simulink model "ScriptDemo"  (R2022b)
settings: configuration reference "TmVcThermal_Configuration_sub" (kept outside this file)
undefined symbols (not defined in the file): aaaa, bbbb, cTmComprCtrl_D_u8HvacFlowTable_db, cTmComprCtrl_D_u8HvacFlowTable_sw, cTmComprCtrl_n_i16ChillCmpIMax, cTmComprCtrl_n_i16ChillCmpIMin, cTmComprCtrl_n_i16ChillCmpIMin666, cTmComprCtrl_n_i16ChillCmpPMax, cTmComprCtrl_n_i16ChillCmpPMin, cTmComprCtrl_n_i16CmpChillCoolRpmKiMax, cTmComprCtrl_n_i16CmpChillCoolRpmKiMin, cTmComprCtrl_n_i16CmpChillCoolRpmKpMax, cTmComprCtrl_n_i16CmpChillCoolRpmKpMin, cTmComprCtrl_n_i16CmpCoolRpmKiMax, cTmComprCtrl_n_i16CmpCoolRpmKiMin, cTmComprCtrl_n_i16CmpCoolRpmKpMax, cTmComprCtrl_n_i16CmpCoolRpmKpMin, cTmComprCtrl_n_i16SM4CmpHeatKiMax, cTmComprCtrl_n_i16SM4CmpHeatKiMin, cTmComprCtrl_n_i16SM4CmpHeatKpMax, cTmComprCtrl_n_i16SM4CmpHeatKpMin, cTmComprCtrl_n_i16SM5CmpHeatKiMax, cTmComprCtrl_n_i16SM5CmpHeatKiMin, cTmComprCtrl_n_i16SM5CmpHeatKpMax, cTmComprCtrl_n_i16SM5CmpHeatKpMin, cTmComprCtrl_n_i16SM6CmpHeatKiMax, cTmComprCtrl_n_i16SM6CmpHeatKiMin, cTmComprCtrl_n_i16SM6CmpHeatKpMax, cTmComprCtrl_n_i16SM6CmpHeatKpMin, cTmComprCtrl_n_u16CmpMaxSpdFanFltLimt, cTmComprCtrl_n_u16CmpMaxSpdLoSidePFltLimt, cTmComprCtrl_n_u16CmpMaxSpdSensorFltLimt, cTmComprCtrl_n_u16CompMinRpm, cTmComprCtrl_n_u16CompRpmIncThres, cTmComprCtrl_t_u16BattCooltFFPeriod, cTmComprCtrl_t_u16BattCooltPIPeriod, cTmComprCtrl_t_u16CmpCoolFFPeriod, cTmComprCtrl_t_u16CmpCoolPIPeriod, cTmComprCtrl_t_u16CoolCmpChillFFPeriod, cTmComprCtrl_t_u16CoolCmpChillPIPeriod, cTmComprCtrl_t_u16SM4CmpHeatFFPeriod, cTmComprCtrl_t_u16SM4CmpHeatPIPeriod, cTmComprCtrl_t_u16SM5CmpHeatFFPeriod, cTmComprCtrl_t_u16SM5CmpHeatPIPeriod, cTmComprCtrl_t_u16SM6CmpHeatFFPeriod, cTmComprCtrl_t_u16SM6CmpHeatPIPeriod, cTmComprCtrl_Te_EvapClearInteg, cTmComprCtrl_Te_i16HpReqTempSaturoffset, cTmComprCtrl_Te_i16SatLpReplaceDiff, cTmComprCtrl_Te_i16SM3BatDiffStartEvapDecOffset, cTmComprCtrl_Te_i16SM3EvapLo, cTmComprCtrl_Te_i16SM3TBatDiffEntEvapDecOffset, cTmComprCtrl_Te_i16SM3TBatDiffEntEvapDecOffsetQuit, cTmComprCtrl_Te_s32ErrCmpChillPIContinueCoolH, cTmComprCtrl_Te_s32ErrCmpChillPIContinueCoolL, cTmComprCtrl_Te_s32ErrCmpPIContinueChillH, cTmComprCtrl_Te_s32ErrCmpPIContinueChillL, cTmComprCtrl_Te_s32ErrCmpPIContinueCoolH, cTmComprCtrl_Te_s32ErrCmpPIContinueCoolL, cTmComprCtrl_Te_s32ErrCmpPIContinueHeatH ... (+398)
libraries: simulink x782, PCMULib x640, simulink_need_slupdate x4
(part 13 of 41)

== system ScriptDemo/Create/createMerge/After/SM2SM22 ==
  note: 1: 非热泵
      | 2：热泵
  sTmSigProces_Te_s32EvapFanReqRamp : Inport  OutDataTypeStr=single
  sTmDiag_D_u8TeEvapFltSt : Inport  Port=2  OutDataTypeStr=uint8
  sTmIn_D_u8HeatPump : Inport  Port=3  OutDataTypeStr=uint8
  sTmSigProces_Te_s32TAmb : Inport  Port=4  OutDataTypeStr=single
  sTmIn_X_s32ClimtRcirc : Inport  Port=5  OutDataTypeStr=single
  sTmComprCtrl_D_u8HvacFlowLevel : Inport  Port=6  OutDataTypeStr=uint8
  sTmSigProces_Te_s32EvapFanFilter : Inport  Port=7  OutDataTypeStr=single
  sTmSigProces_Te_s32SatLp : Inport  Port=8  OutDataTypeStr=single
  xTmComprCtrl_B_CompOnReqCompOn : Inport  Port=9  OutDataTypeStr=boolean
  yTmRefriModeMgr_B_CoolModeInCycle : Inport  Port=10  OutDataTypeStr=boolean
  yTmRefriModeMgr_B_CoolOCRMode : Inport  Port=11  OutDataTypeStr=boolean
  sTmSigProces_Pw_i16ReqPwrForCool : Inport  Port=12  OutDataTypeStr=int16
  Action Port : ActionPort
  1-D Lookup Table : Lookup_n-D  NumberOfTableDimensions=1  BreakpointsForDimension1=tTmComprCtrl_n_i16CmpCoolRpmKiMin_X  BreakpointsForDimension1DataTypeStr=Inherit: Inherit from 'Breakpoint data'  Table=tTmComprCtrl_n_i16CmpCoolRpmKiMin  TableDataTypeStr=Inherit: Inherit from 'Table data'  ExtrapMethod=Clip  InternalRulePriority=Speed  OutDataTypeStr=Inherit: Inherit via back propagation  RndMeth=Simplest  InputSameDT=off
  1-D Lookup Table1 : Lookup_n-D  NumberOfTableDimensions=1  BreakpointsForDimension1=tTmComprCtrl_n_i16CmpCoolRpmKiMax_X  BreakpointsForDimension1DataTypeStr=Inherit: Inherit from 'Breakpoint data'  Table=tTmComprCtrl_n_i16CmpCoolRpmKiMax  TableDataTypeStr=Inherit: Inherit from 'Table data'  ExtrapMethod=Clip  InternalRulePriority=Speed  OutDataTypeStr=Inherit: Inherit via back propagation  RndMeth=Simplest  InputSameDT=off
  Compare To Constant1 : simulink/Logic and Bit Operations/Compare To Constant  relop===  const=2  OutDataTypeStr=boolean
  Constant : Constant  Value=cTmComprCtrl_n_i16CmpCoolRpmKpMax  OutDataTypeStr=int16
  Constant3 : Constant  Value=cTmComprCtrl_t_u16CmpCoolPIPeriod  OutDataTypeStr=uint16
  Constant4 : Constant  Value=cTmComprCtrl_n_i16CmpCoolRpmKpMin  OutDataTypeStr=int16
  Constant5 : Constant  Value=cTmComprCtrl_Te_s32ErrCmpPIContinueCoolH  OutDataTypeStr=single
  Constant6 : Constant  Commented=on  Value=cTmComprCtrl_n_i16CmpCoolRpmKiMax  OutDataTypeStr=int16
  Constant7 : Constant  Value=cTmComprCtrl_Te_s32ErrCmpPIContinueCoolL  OutDataTypeStr=single
  Constant8 : Constant  Commented=on  Value=cTmComprCtrl_n_i16CmpCoolRpmKiMin  OutDataTypeStr=int16
  Constant9 : Constant  Value=cTmComprCtrl_n_u16CompMinRpm
  ID26239_SM2Error : Subsystem
  ID26267_SM2FF : Subsystem
  Logical Operator : Logic  AllPortsSameDT=off  OutDataTypeStr=boolean
  Logical Operator2 : Logic  Operator=NOT  AllPortsSameDT=off  OutDataTypeStr=boolean
  SM2FFEnable : Subsystem
  SM2_Ki : Subsystem
  SM2_Kp : Subsystem
  rSM2SM22_n_u16DisOverrideValue : Outport  OutDataTypeStr=uint16
  rSM2SM22_t_u16PIPeriod : Outport  Port=2  OutDataTypeStr=uint16
  rSM2SM22_Te_s32UpErrStop : Outport  Port=3  OutDataTypeStr=single
  rSM2SM22_n_u16ComprRpmFF : Outport  Port=4  OutDataTypeStr=uint16
  rSM2SM22_n_u16ComprRpmKp : Outport  Port=5  OutDataTypeStr=uint16
  rSM2SM22_n_u16ComprRpmKi : Outport  Port=6  OutDataTypeStr=uint16
  rSM2SM22_Te_s32LowErrStop : Outport  Port=7  OutDataTypeStr=single
  rSM2SM22_n_i16KpUpLimit : Outport  Port=8  OutDataTypeStr=int16
  rSM2SM22_n_i16KpLowLimit : Outport  Port=9  OutDataTypeStr=int16
  rSM2SM22_n_i16KiUpLimit : Outport  Port=10  OutDataTypeStr=int16
  rSM2SM22_n_i16KiLowLimit : Outport  Port=11  OutDataTypeStr=int16
  xSM2SM22_B_Enable : Outport  Port=12  OutDataTypeStr=boolean
  rSM2SM22_Te_s32TempError : Outport  Port=13  OutDataTypeStr=single
  wires:
  sTmSigProces_Te_s32EvapFanReqRamp/1 -> [sTmSigProces_Te_s32EvapFanReqRamp]
  sTmDiag_D_u8TeEvapFltSt/1 -> [sTmDiag_D_u8TeEvapFltSt]
  sTmIn_D_u8HeatPump/1 -> [sTmIn_D_u8HeatPump]
  sTmSigProces_Te_s32TAmb/1 -> [sTmSigProces_Te_s32TAmb]
  sTmIn_X_s32ClimtRcirc/1 -> [sTmIn_X_s32ClimtRcirc]
  sTmComprCtrl_D_u8HvacFlowLevel/1 -> [sTmComprCtrl_D_u8HvacFlowLevel]
  sTmSigProces_Te_s32EvapFanFilter/1 -> [sTmSigProces_Te_s32EvapFanFilter]
  sTmSigProces_Te_s32SatLp/1 -> [sTmSigProces_Te_s32SatLp]
  xTmComprCtrl_B_CompOnReqCompOn/1 -> [xTmComprCtrl_B_CompOnReqCompOn]
  yTmRefriModeMgr_B_CoolModeInCycle/1 -> [yTmRefriModeMgr_B_CoolModeInCycle]
  [sTmSigProces_Te_s32EvapFanReqRamp] -> ID26267_SM2FF/1(sTmSigProces_Te_s32EvapFanReqRamp)
  [sTmSigProces_Te_s32TAmb] -> ID26267_SM2FF/2(sTmSigProces_Te_s32TAmb)
  [sTmIn_X_s32ClimtRcirc] -> ID26267_SM2FF/3(sTmIn_X_s32ClimtRcirc)
  [sTmComprCtrl_D_u8HvacFlowLevel] -> ID26267_SM2FF/4(sTmComprCtrl_D_u8HvacFlowLevel)
  [rTmComprCtrl_Te_s32TempError] -> SM2_Ki/1(rTmComprCtrl_Te_s32TempError)
  [sTmSigProces_Te_s32TAmb] -> SM2_Ki/2(sTmSigProces_Te_s32TAmb)
  [sTmIn_X_s32ClimtRcirc] -> SM2_Ki/3(sTmIn_X_s32ClimtRcirc)
  [sTmComprCtrl_D_u8HvacFlowLevel] -> SM2_Ki/4(sTmComprCtrl_D_u8HvacFlowLevel)
  [rTmComprCtrl_Te_s32TempError] -> SM2_Kp/1(rTmComprCtrl_Te_s32TempError)
  [sTmSigProces_Te_s32TAmb] -> SM2_Kp/2(sTmSigProces_Te_s32TAmb)
  [sTmIn_X_s32ClimtRcirc] -> SM2_Kp/3(sTmIn_X_s32ClimtRcirc)
  [sTmComprCtrl_D_u8HvacFlowLevel] -> SM2_Kp/4(sTmComprCtrl_D_u8HvacFlowLevel)
  [sTmSigProces_Te_s32EvapFanReqRamp] -> ID26239_SM2Error/1(sTmSigProces_Te_s32EvapFanReqRamp)
  [sTmDiag_D_u8TeEvapFltSt] -> ID26239_SM2Error/2(sTmDiag_D_u8TeEvapFltSt)
  [sTmSigProces_Te_s32EvapFanFilter] -> ID26239_SM2Error/3(sTmSigProces_Te_s32EvapFanFilter)
  [sTmSigProces_Te_s32SatLp] -> ID26239_SM2Error/4(sTmSigProces_Te_s32SatLp)
  SM2FFEnable/1(SM2FFEnable_B_SM2FFEnable) -> [SM2FFEnable_B_SM2FFEnable]
  [xTmComprCtrl_B_CompOnReqCompOn] -> SM2FFEnable/1(xTmComprCtrl_B_CompOnReqCompOn)
  [SM2FFEnable_B_SM2FFEnable] -> ID26267_SM2FF/Enable
  ID26239_SM2Error/1(rTmComprCtrl_Te_s32TempError) -> [rTmComprCtrl_Te_s32TempError]
  ID26267_SM2FF/1(SM2FF) -> [rTmComprCtrl_n_u16ComprRpmFF]
  SM2_Kp/1(SM2Kp) -> [rTmComprCtrl_n_u16ComprRpmKp]
  SM2_Ki/1(SM2Ki) -> [rTmComprCtrl_n_u16ComprRpmKi]
  Constant9/1 -> [rTmComprCtrl_n_u16DisOverrideValue]
  Constant5/1 -> [rTmComprCtrl_Te_s32UpErrStop]
  Constant7/1 -> [rTmComprCtrl_Te_s32LowErrStop]
  Constant3/1 -> [rTmComprCtrl_t_u16PIPeriod]
  Constant/1 -> [rTmComprCtrl_n_i16KpUpLimit]
  Logical Operator/1 -> Logical Operator2/1
  [sTmIn_D_u8HeatPump] -> Compare To Constant1/1
  Compare To Constant1/1 -> Logical Operator/1
  [yTmRefriModeMgr_B_CoolModeInCycle] -> Logical Operator/2
  Logical Operator2/1 -> [xTmComprCtrl_B_Enable]
  [yTmRefriModeMgr_B_CoolOCRMode] -> ID26239_SM2Error/5(yTmRefriModeMgr_B_CoolOCRMode)
  yTmRefriModeMgr_B_CoolOCRMode/1 -> [yTmRefriModeMgr_B_CoolOCRMode]
  [sTmIn_D_u8HeatPump] -> ID26267_SM2FF/5(sTmIn_D_u8HeatPump)
  [sTmSigProces_Pw_i16ReqPwrForCool] -> 1-D Lookup Table/1, 1-D Lookup Table1/1
  Constant4/1 -> [rTmComprCtrl_n_i16KpLowLimit]
  1-D Lookup Table1/1 -> [rTmComprCtrl_n_i16KiUpLimit]
  1-D Lookup Table/1 -> [rTmComprCtrl_n_i16KiLowLimit]
  sTmSigProces_Pw_i16ReqPwrForCool/1 -> [sTmSigProces_Pw_i16ReqPwrForCool]
  [rTmComprCtrl_n_u16DisOverrideValue] -> rSM2SM22_n_u16DisOverrideValue/1
  [rTmComprCtrl_t_u16PIPeriod] -> rSM2SM22_t_u16PIPeriod/1
  [rTmComprCtrl_Te_s32UpErrStop] -> rSM2SM22_Te_s32UpErrStop/1
  [rTmComprCtrl_n_u16ComprRpmFF] -> rSM2SM22_n_u16ComprRpmFF/1
  [rTmComprCtrl_n_u16ComprRpmKp] -> rSM2SM22_n_u16ComprRpmKp/1
  [rTmComprCtrl_n_u16ComprRpmKi] -> rSM2SM22_n_u16ComprRpmKi/1
  [rTmComprCtrl_Te_s32LowErrStop] -> rSM2SM22_Te_s32LowErrStop/1
  [rTmComprCtrl_n_i16KpUpLimit] -> rSM2SM22_n_i16KpUpLimit/1
  [rTmComprCtrl_n_i16KpLowLimit] -> rSM2SM22_n_i16KpLowLimit/1
  [rTmComprCtrl_n_i16KiUpLimit] -> rSM2SM22_n_i16KiUpLimit/1
  [rTmComprCtrl_n_i16KiLowLimit] -> rSM2SM22_n_i16KiLowLimit/1
  [xTmComprCtrl_B_Enable] -> xSM2SM22_B_Enable/1
  [rTmComprCtrl_Te_s32TempError] -> rSM2SM22_Te_s32TempError/1

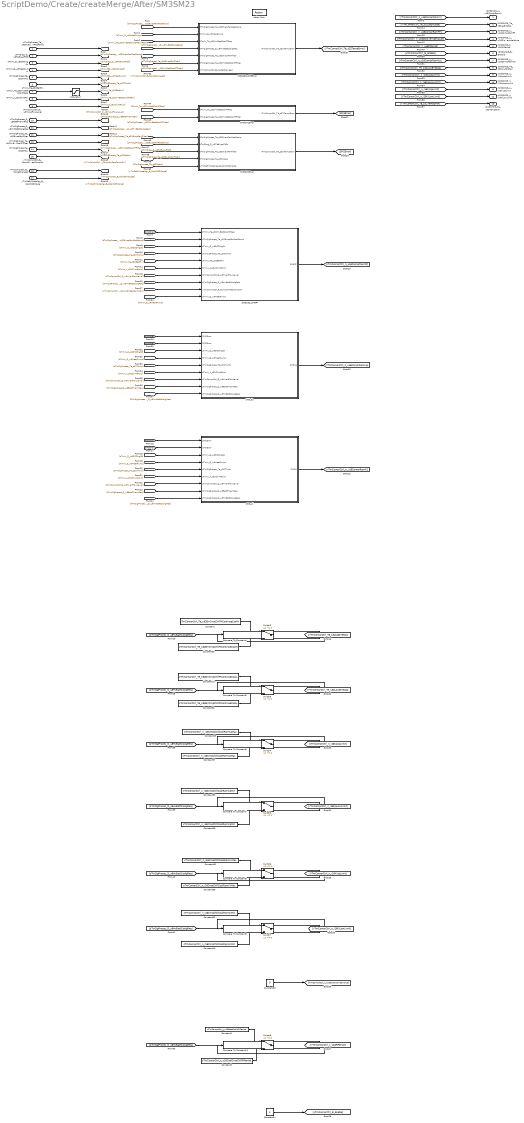
== system ScriptDemo/Create/createMerge/After/SM3SM23 ==
  sTmSigProces_Te_s32EvapFanReqRamp : Inport  OutDataTypeStr=single
  sTmDiag_D_u8TeEvapFltSt : Inport  Port=2  OutDataTypeStr=uint8
  sTmIn_D_u8DCChrgSt : Inport  Port=3  OutDataTypeStr=uint8
  sTmIn_D_u8HeatPump : Inport  Port=4  OutDataTypeStr=uint8
  sTmSigProces_Te_s32TAmb : Inport  Port=5  OutDataTypeStr=single
  sTmIn_Te_s32BattHv : Inport  Port=6  OutDataTypeStr=single
  sTmIn_Te_s32HvBattCooltTReq : Inport  Port=7  OutDataTypeStr=single
  sTmIn_X_s32ClimtRcirc : Inport  Port=8  OutDataTypeStr=single
  sTmComprCtrl_D_u8HvacFlowLevel : Inport  Port=9  OutDataTypeStr=uint8
  sTmSigProces_D_u8BattThermReq : Inport  Port=10  OutDataTypeStr=uint8
  sTmSigProces_D_u8HvBattCoolgReq : Inport  Port=11  OutDataTypeStr=uint8
  sTmSigProces_Te_s32EvapFanFilter : Inport  Port=12  OutDataTypeStr=single
  sTmSigProces_Te_s32HvBattCooltTFilter : Inport  Port=13  OutDataTypeStr=single
  sTmSigProces_Te_s32SatLp : Inport  Port=14  OutDataTypeStr=single
  xTmComprCtrl_B_CompOnReqCompOn : Inport  Port=15  OutDataTypeStr=boolean
  xTmComprCtrl_B_ModeChanged : Inport  Port=16  OutDataTypeStr=boolean
  yTmRefriModeMgr_B_CoolOCRMode : Inport  Port=17  OutDataTypeStr=boolean
  Action Port : ActionPort
  Compare To Constant{4..9,11} (7 alike) : simulink/Logic and Bit Operations/Compare To Constant  relop===  const=3  OutDataTypeStr=boolean
  Constant : Constant  Value=cTmComprCtrl_Te_s32ErrCmpChillPIContinueCoolH  OutDataTypeStr=single
  Constant1 : Constant  Value=cTmComprCtrl_t_u16BattCooltPIPeriod  OutDataTypeStr=uint16
  Constant13 : Constant  Value=cTmComprCtrl_Te_s32ErrCmpChillPIContinueCoolL  OutDataTypeStr=single
  Constant2 : Constant  Value=cTmComprCtrl_t_u16CoolCmpChillPIPeriod  OutDataTypeStr=uint16
  Constant29 : Constant  Value=cTmComprCtrl_n_i16CmpChillCoolRpmKpMax
  Constant30 : Constant  Value=cTmComprCtrl_n_i16CmpChillCoolRpmKpMin
  Constant31 : Constant  Value=cTmComprCtrl_n_i16CmpChillCoolRpmKiMax
  Constant32 : Constant  Value=cTmComprCtrl_n_i16CmpChillCoolRpmKiMin
  Constant33 : Constant  Value=0  OutDataTypeStr=uint16
  Constant34 : Constant  OutDataTypeStr=boolean
  Constant35 : Constant  Value=cTmComprCtrl_Te_s32ErrCmpChillPIContinueCoolH  OutDataTypeStr=single
  Constant36 : Constant  Value=cTmComprCtrl_Te_s32ErrCmpChillPIContinueCoolL  OutDataTypeStr=single
  Constant37 : Constant  Value=cTmComprCtrl_n_i16CmpChillCoolRpmKpMax
  Constant38 : Constant  Value=cTmComprCtrl_n_i16CmpChillCoolRpmKpMin
  Constant39 : Constant  Value=cTmComprCtrl_n_i16CmpChillCoolRpmKiMax
  Constant40 : Constant  Value=cTmComprCtrl_n_i16CmpChillCoolRpmKiMin
  ID26262_SM3FF : Subsystem
  ID26263_SM3Error : Subsystem
  SM3SM1Error : Subsystem
  SM3SM2Error : Subsystem
  SM3_Ki : Subsystem
  SM3_Kp : Subsystem
  Saturation : Saturate  UpperLimit=40  LowerLimit=12
  Switch{2..7,9} (7 alike) : Switch  Criteria=u2 ~= 0  SaturateOnIntegerOverflow=off  InputSameDT=off
  rSM3SM23_n_u16ComprRpmKi : Outport  OutDataTypeStr=uint16
  rSM3SM23_Te_s32UpErrStop : Outport  Port=2  OutDataTypeStr=single
  rSM3SM23_n_u16ComprRpmFF : Outport  Port=3  OutDataTypeStr=uint16
  rSM3SM23_n_u16DisOverrideValue : Outport  Port=4  OutDataTypeStr=uint16
  rSM3SM23_t_u16PIPeriod : Outport  Port=5  OutDataTypeStr=uint16
  xSM3SM23_B_Enable : Outport  Port=6  OutDataTypeStr=boolean
  rSM3SM23_n_u16ComprRpmKp : Outport  Port=7  OutDataTypeStr=uint16
  rSM3SM23_Te_s32LowErrStop : Outport  Port=8  OutDataTypeStr=single
  rSM3SM23_n_i16KpUpLimit : Outport  Port=9  OutDataTypeStr=int16
  rSM3SM23_n_i16KpLowLimit : Outport  Port=10  OutDataTypeStr=int16
  rSM3SM23_n_i16KiUpLimit : Outport  Port=11  OutDataTypeStr=int16
  rSM3SM23_n_i16KiLowLimit : Outport  Port=12  OutDataTypeStr=int16
  rSM3SM23_Te_s32TempError : Outport  Port=13  OutDataTypeStr=single
  wires:
  ID26263_SM3Error/1(rTmComprCtrl_Te_s32TempError) -> [rTmComprCtrl_Te_s32TempError]
  [sTmIn_Te_s32HvBattCooltTReq] -> SM3SM1Error/1(sTmIn_Te_s32HvBattCooltTReq)
  [sTmSigProces_Te_s32HvBattCooltTFilter] -> SM3SM1Error/2(sTmSigProces_Te_s32HvBattCooltTFilter)
  [sTmDiag_D_u8TeEvapFltSt] -> SM3SM2Error/2(sTmDiag_D_u8TeEvapFltSt)
  [sTmSigProces_Te_s32EvapFanFilter] -> SM3SM2Error/3(sTmSigProces_Te_s32EvapFanFilter)
  [sTmSigProces_Te_s32SatLp] -> SM3SM2Error/4(sTmSigProces_Te_s32SatLp)
  SM3SM2Error/1(rTmComprCtrl_Te_s32TempError) -> [SM2Error]
  [sTmSigProces_Te_s32EvapFanReqRamp] -> SM3SM2Error/1(sTmSigProces_Te_s32EvapFanReqRamp)
  [SM1Error] -> SM3_Ki/1(SM1Error)
  [SM2Error] -> SM3_Ki/2(SM2Error)
  [sTmIn_D_u8DCChrgSt] -> SM3_Ki/3(sTmIn_D_u8DCChrgSt)
  [sTmIn_D_u8HeatPump] -> SM3_Ki/4(sTmIn_D_u8HeatPump)
  [sTmSigProces_Te_s32TAmb] -> SM3_Ki/5(sTmSigProces_Te_s32TAmb)
  [sTmIn_X_s32ClimtRcirc] -> SM3_Ki/6(sTmIn_X_s32ClimtRcirc)
  [sTmComprCtrl_D_u8HvacFlowLevel] -> SM3_Ki/7(sTmComprCtrl_D_u8HvacFlowLevel)
  [sTmSigProces_D_u8BattThermReq] -> SM3_Ki/8(sTmSigProces_D_u8BattThermReq)
  [sTmSigProces_D_u8HvBattCoolgReq] -> SM3_Ki/9(sTmSigProces_D_u8HvBattCoolgReq)
  [SM1Error] -> SM3_Kp/1(SM1Error)
  [SM2Error] -> SM3_Kp/2(SM2Error)
  [sTmIn_D_u8DCChrgSt] -> SM3_Kp/3(sTmIn_D_u8DCChrgSt)
  [sTmIn_D_u8HeatPump] -> SM3_Kp/4(sTmIn_D_u8HeatPump)
  [sTmSigProces_Te_s32TAmb] -> SM3_Kp/5(sTmSigProces_Te_s32TAmb)
  [sTmIn_X_s32ClimtRcirc] -> SM3_Kp/6(sTmIn_X_s32ClimtRcirc)
  [sTmComprCtrl_D_u8HvacFlowLevel] -> SM3_Kp/7(sTmComprCtrl_D_u8HvacFlowLevel)
  [sTmSigProces_D_u8BattThermReq] -> SM3_Kp/8(sTmSigProces_D_u8BattThermReq)
  [sTmSigProces_D_u8HvBattCoolgReq] -> SM3_Kp/9(sTmSigProces_D_u8HvBattCoolgReq)
  sTmSigProces_Te_s32EvapFanReqRamp/1 -> [sTmSigProces_Te_s32EvapFanReqRamp]
  sTmDiag_D_u8TeEvapFltSt/1 -> [sTmDiag_D_u8TeEvapFltSt]
  sTmIn_D_u8DCChrgSt/1 -> [sTmIn_D_u8DCChrgSt]
  sTmIn_D_u8HeatPump/1 -> [sTmIn_D_u8HeatPump]
  sTmSigProces_Te_s32TAmb/1 -> [sTmSigProces_Te_s32TAmb]
  sTmIn_Te_s32BattHv/1 -> [sTmIn_Te_s32BattHv]
  sTmIn_Te_s32HvBattCooltTReq/1 -> Saturation/1
  sTmIn_X_s32ClimtRcirc/1 -> [sTmIn_X_s32ClimtRcirc]
  sTmComprCtrl_D_u8HvacFlowLevel/1 -> [sTmComprCtrl_D_u8HvacFlowLevel]
  sTmSigProces_D_u8BattThermReq/1 -> [sTmSigProces_D_u8BattThermReq]
  sTmSigProces_D_u8HvBattCoolgReq/1 -> [sTmSigProces_D_u8HvBattCoolgReq]
  sTmSigProces_Te_s32EvapFanFilter/1 -> [sTmSigProces_Te_s32EvapFanFilter]
  sTmSigProces_Te_s32HvBattCooltTFilter/1 -> [sTmSigProces_Te_s32HvBattCooltTFilter]
  sTmSigProces_Te_s32SatLp/1 -> [sTmSigProces_Te_s32SatLp]
  xTmComprCtrl_B_CompOnReqCompOn/1 -> [xTmComprCtrl_B_CompOnReqCompOn]
  [SM1Error] -> ID26262_SM3FF/1(sTmIn_Te_s32HvBattCooltTReq)
  [sTmSigProces_Te_s32EvapFanReqRamp] -> ID26262_SM3FF/2(sTmSigProces_Te_s32EvapFanReqRamp)
  [sTmIn_D_u8DCChrgSt] -> ID26262_SM3FF/3(sTmIn_D_u8DCChrgSt)
  [sTmSigProces_Te_s32TAmb] -> ID26262_SM3FF/4(sTmSigProces_Te_s32TAmb)
  [sTmIn_Te_s32BattHv] -> ID26262_SM3FF/5(sTmIn_Te_s32BattHv)
  [sTmIn_X_s32ClimtRcirc] -> ID26262_SM3FF/6(sTmIn_X_s32ClimtRcirc)
  [sTmComprCtrl_D_u8HvacFlowLevel] -> ID26262_SM3FF/7(sTmComprCtrl_D_u8HvacFlowLevel)
  [sTmSigProces_D_u8HvBattCoolgReq] -> ID26262_SM3FF/8(sTmSigProces_D_u8HvBattCoolgReq)
  SM3SM1Error/1(rTmComprCtrl_Te_s32TempError) -> [SM1Error]
  [sTmSigProces_Te_s32EvapFanReqRamp] -> ID26263_SM3Error/1(sTmSigProces_Te_s32EvapFanReqRamp)
  [sTmIn_D_u8HeatPump] -> ID26263_SM3Error/2(sTmIn_D_u8HeatPump)
  [sTmIn_Te_s32HvBattCooltTReq] -> ID26263_SM3Error/3(sTmIn_Te_s32HvBattCooltTReq)
  [sTmSigProces_D_u8HvBattCoolgReq] -> ID26263_SM3Error/4(sTmSigProces_D_u8HvBattCoolgReq)
  [sTmSigProces_Te_s32EvapFanFilter] -> ID26263_SM3Error/5(sTmSigProces_Te_s32EvapFanFilter)
  [sTmSigProces_Te_s32HvBattCooltTFilter] -> ID26263_SM3Error/6(sTmSigProces_Te_s32HvBattCooltTFilter)
  [xTmComprCtrl_B_CompOnReqCompOn] -> ID26262_SM3FF/9(xTmComprCtrl_B_CompOnReqCompOn)
  ID26262_SM3FF/1(SM3FF) -> [rTmComprCtrl_n_u16ComprRpmFF]
  SM3_Kp/1(SM3Kp) -> [rTmComprCtrl_n_u16ComprRpmKp]
  [sTmSigProces_D_u8HvBattCoolgReq] -> Compare To Constant4/1
  Compare To Constant4/1 -> Switch2/2
  Switch2/1 -> [rTmComprCtrl_Te_s32UpErrStop]
  [sTmSigProces_D_u8HvBattCoolgReq] -> Compare To Constant5/1
  Switch3/1 -> [rTmComprCtrl_Te_s32LowErrStop]
  Compare To Constant5/1 -> Switch3/2
  Compare To Constant6/1 -> Switch4/2
  Switch4/1 -> [rTmComprCtrl_n_i16KpUpLimit]
  [sTmSigProces_D_u8HvBattCoolgReq] -> Compare To Constant6/1
  [sTmSigProces_D_u8HvBattCoolgReq] -> Compare To Constant7/1
  Switch5/1 -> [rTmComprCtrl_n_i16KpLowLimit]
  Compare To Constant7/1 -> Switch5/2
  Compare To Constant11/1 -> Switch9/2
  Switch7/1 -> [rTmComprCtrl_n_i16KiLowLimit]
  Switch9/1 -> [rTmComprCtrl_t_u16PIPeriod]
  Compare To Constant9/1 -> Switch7/2
  [sTmSigProces_D_u8HvBattCoolgReq] -> Compare To Constant11/1
  [sTmSigProces_D_u8HvBattCoolgReq] -> Compare To Constant9/1
  [sTmSigProces_D_u8HvBattCoolgReq] -> Compare To Constant8/1
  Switch6/1 -> [rTmComprCtrl_n_i16KiUpLimit]
  Constant33/1 -> [rTmComprCtrl_n_u16DisOverrideValue]
  Compare To Constant8/1 -> Switch6/2
  Constant34/1 -> [xTmComprCtrl_B_Enable]
  Constant2/1 -> Switch9/3
  Constant1/1 -> Switch9/1
  Constant/1 -> Switch2/1
  Constant13/1 -> Switch3/1
  Constant29/1 -> Switch4/1
  Constant30/1 -> Switch5/1
  Constant31/1 -> Switch6/1
  Constant32/1 -> Switch7/1
  Constant35/1 -> Switch2/3
  Constant36/1 -> Switch3/3
  Constant37/1 -> Switch4/3
  Constant38/1 -> Switch5/3
  Constant39/1 -> Switch6/3
  Constant40/1 -> Switch7/3
  SM3_Ki/1(SM3Ki) -> [rTmComprCtrl_n_u16ComprRpmKi]
  [xTmComprCtrl_B_ModeChanged] -> ID26263_SM3Error/7(xTmComprCtrl_B_ModeChanged)
  xTmComprCtrl_B_ModeChanged/1 -> [xTmComprCtrl_B_ModeChanged]
  [yTmRefriModeMgr_B_CoolOCRMode] -> SM3SM2Error/5(yTmRefriModeMgr_B_CoolOCRMode)
  yTmRefriModeMgr_B_CoolOCRMode/1 -> [yTmRefriModeMgr_B_CoolOCRMode]
  Saturation/1 -> [sTmIn_Te_s32HvBattCooltTReq]
  [sTmIn_D_u8HeatPump] -> ID26262_SM3FF/10(sTmIn_D_u8HeatPump)
  [rTmComprCtrl_n_u16ComprRpmKi] -> rSM3SM23_n_u16ComprRpmKi/1
  [rTmComprCtrl_Te_s32UpErrStop] -> rSM3SM23_Te_s32UpErrStop/1
  [rTmComprCtrl_n_u16ComprRpmFF] -> rSM3SM23_n_u16ComprRpmFF/1
  [rTmComprCtrl_n_u16DisOverrideValue] -> rSM3SM23_n_u16DisOverrideValue/1
  [rTmComprCtrl_t_u16PIPeriod] -> rSM3SM23_t_u16PIPeriod/1
  [xTmComprCtrl_B_Enable] -> xSM3SM23_B_Enable/1
  [rTmComprCtrl_n_u16ComprRpmKp] -> rSM3SM23_n_u16ComprRpmKp/1
  [rTmComprCtrl_Te_s32LowErrStop] -> rSM3SM23_Te_s32LowErrStop/1
  [rTmComprCtrl_n_i16KpUpLimit] -> rSM3SM23_n_i16KpUpLimit/1
  [rTmComprCtrl_n_i16KpLowLimit] -> rSM3SM23_n_i16KpLowLimit/1
  [rTmComprCtrl_n_i16KiUpLimit] -> rSM3SM23_n_i16KiUpLimit/1
  [rTmComprCtrl_n_i16KiLowLimit] -> rSM3SM23_n_i16KiLowLimit/1
  [rTmComprCtrl_Te_s32TempError] -> rSM3SM23_Te_s32TempError/1

== system ScriptDemo/Create/createMerge/After/SM4 ==
  sTmSigProces_Te_s32HeatrAirTReqRamp : Inport  OutDataTypeStr=single
  sTmSigProces_Te_s32HvacHexAirTFilter : Inport  Port=2  OutDataTypeStr=single
  sTmSigProces_Te_s32TAmb : Inport  Port=3  OutDataTypeStr=single
  sTmSigProces_Te_s32SatHp : Inport  Port=4  OutDataTypeStr=single
  sTmComprCtrl_D_u8HvacFlowLevel : Inport  Port=5  OutDataTypeStr=uint8
  xTmComprCtrl_B_CompOnReqCompOn : Inport  Port=6  OutDataTypeStr=boolean
  yTmHvchCtrl_B_HpcPtcEnad : Inport  Port=7  OutDataTypeStr=boolean
  sTmSigProces_Te_s32TempInlet : Inport  Port=8  OutDataTypeStr=single
  yTmRefriModeMgr_B_HeatModeInCycle : Inport  Port=9  OutDataTypeStr=boolean
  Action Port : ActionPort
  Constant : Constant  Value=cTmComprCtrl_n_i16SM4CmpHeatKpMax  OutDataTypeStr=int16
  Constant15 : Constant  Value=cTmComprCtrl_Te_s32ErrCmpPIContinueHeatL  OutDataTypeStr=single
  Constant16 : Constant  Value=cTmComprCtrl_n_i16SM4CmpHeatKiMin  OutDataTypeStr=int16
  Constant2 : Constant  Value=cTmComprCtrl_n_u16CompMinRpm
  Constant6 : Constant  Value=cTmComprCtrl_t_u16SM4CmpHeatPIPeriod  OutDataTypeStr=uint16
  Constant7 : Constant  Value=cTmComprCtrl_n_i16SM4CmpHeatKpMin  OutDataTypeStr=int16
  Constant8 : Constant  Value=cTmComprCtrl_Te_s32ErrCmpPIContinueHeatH  OutDataTypeStr=single
  Constant9 : Constant  Value=cTmComprCtrl_n_i16SM4CmpHeatKiMax  OutDataTypeStr=int16
  ID26259_SM4Error : Subsystem
  ID26297_SM4FF : Subsystem
  Logical Operator : Logic  Operator=NOT  AllPortsSameDT=off  OutDataTypeStr=boolean
  SM24FFEnable : Subsystem
  SM4_Ki : Subsystem
  SM4_Kp : Subsystem
  rSM4_n_u16DisOverrideValue : Outport  OutDataTypeStr=uint16
  rSM4_t_u16PIPeriod : Outport  Port=2  OutDataTypeStr=uint16
  rSM4_Te_s32UpErrStop : Outport  Port=3  OutDataTypeStr=single
  rSM4_n_u16ComprRpmFF : Outport  Port=4  OutDataTypeStr=uint16
  rSM4_n_u16ComprRpmKp : Outport  Port=5  OutDataTypeStr=uint16
  rSM4_Te_s32LowErrStop : Outport  Port=6  OutDataTypeStr=single
  rSM4_n_i16KpUpLimit : Outport  Port=7  OutDataTypeStr=int16
  rSM4_n_i16KpLowLimit : Outport  Port=8  OutDataTypeStr=int16
  rSM4_n_i16KiUpLimit : Outport  Port=9  OutDataTypeStr=int16
  rSM4_n_i16KiLowLimit : Outport  Port=10  OutDataTypeStr=int16
  xSM4_B_Enable : Outport  Port=11  OutDataTypeStr=boolean
  rSM4_n_u16ComprRpmKi : Outport  Port=12  OutDataTypeStr=uint16
  rSM4_Te_s32TempError : Outport  Port=13  OutDataTypeStr=single
  wires:
  ID26259_SM4Error/1(rTmComprCtrl_Te_s32TempError) -> [rTmComprCtrl_Te_s32TempError]
  [sTmSigProces_Te_s32SatHp] -> ID26259_SM4Error/1(sTmSigProces_Te_s32SatHp)
  [yTmHvchCtrl_B_HpcPtcEnad] -> ID26259_SM4Error/2(yTmHvchCtrl_B_HpcPtcEnad)
  [sTmSigProces_Te_s32HeatrAirTReqRamp] -> ID26259_SM4Error/3(sTmSigProces_Te_s32HeatrAirTReqRamp)
  [sTmSigProces_Te_s32HvacHexAirTFilter] -> ID26259_SM4Error/4(sTmSigProces_Te_s32HvacHexAirTFilter)
  sTmSigProces_Te_s32HeatrAirTReqRamp/1 -> [sTmSigProces_Te_s32HeatrAirTReqRamp]
  sTmSigProces_Te_s32HvacHexAirTFilter/1 -> [sTmSigProces_Te_s32HvacHexAirTFilter]
  sTmSigProces_Te_s32TAmb/1 -> [sTmSigProces_Te_s32TAmb]
  sTmSigProces_Te_s32SatHp/1 -> [sTmSigProces_Te_s32SatHp]
  sTmComprCtrl_D_u8HvacFlowLevel/1 -> [sTmComprCtrl_D_u8HvacFlowLevel]
  xTmComprCtrl_B_CompOnReqCompOn/1 -> [xTmComprCtrl_B_CompOnReqCompOn]
  yTmHvchCtrl_B_HpcPtcEnad/1 -> [yTmHvchCtrl_B_HpcPtcEnad]
  [xTmComprCtrl_B_CompOnReqCompOn] -> SM24FFEnable/1(xTmComprCtrl_B_CompOnReqCompOn)
  SM24FFEnable/1(SM4FFEnable_B_SM4FFEnable) -> [SM4FFEnable_B_SM4FFEnable]
  [SM4FFEnable_B_SM4FFEnable] -> ID26297_SM4FF/Enable
  Logical Operator/1 -> [xTmComprCtrl_B_Enable]
  Constant2/1 -> [rTmComprCtrl_n_u16DisOverrideValue]
  Constant6/1 -> [rTmComprCtrl_t_u16PIPeriod]
  Constant15/1 -> [rTmComprCtrl_Te_s32LowErrStop]
  Constant/1 -> [rTmComprCtrl_n_i16KpUpLimit]
  Constant8/1 -> [rTmComprCtrl_Te_s32UpErrStop]
  Constant7/1 -> [rTmComprCtrl_n_i16KpLowLimit]
  Constant16/1 -> [rTmComprCtrl_n_i16KiLowLimit]
  Constant9/1 -> [rTmComprCtrl_n_i16KiUpLimit]
  ID26297_SM4FF/1(SM4FF) -> [rTmComprCtrl_n_u16ComprRpmFF]
  SM4_Kp/1(SM4Kp) -> [rTmComprCtrl_n_u16ComprRpmKp]
  SM4_Ki/1(SM4Ki) -> [rTmComprCtrl_n_u16ComprRpmKi]
  sTmSigProces_Te_s32TempInlet/1 -> [sTmSigProces_Te_s32TempInlet]
  [sTmComprCtrl_D_u8HvacFlowLevel] -> ID26297_SM4FF/1(sTmComprCtrl_D_u8HvacFlowLevel)
  [sTmSigProces_Te_s32TempInlet] -> ID26297_SM4FF/2(sTmSigProces_Te_s32TempInlet)
  [sTmSigProces_Te_s32HeatrAirTReqRamp] -> ID26297_SM4FF/3(sTmSigProces_Te_s32HeatrAirTReqRamp)
  [sTmSigProces_Te_s32TAmb] -> ID26297_SM4FF/4(sTmSigProces_Te_s32TAmb)
  [sTmComprCtrl_D_u8HvacFlowLevel] -> SM4_Ki/1(sTmComprCtrl_D_u8HvacFlowLevel)
  [sTmSigProces_Te_s32TAmb] -> SM4_Ki/2(sTmSigProces_Te_s32TAmb)
  [rTmComprCtrl_Te_s32TempError] -> SM4_Ki/3(rTmComprCtrl_Te_s32TempError)
  [sTmComprCtrl_D_u8HvacFlowLevel] -> SM4_Kp/1(sTmComprCtrl_D_u8HvacFlowLevel)
  [sTmSigProces_Te_s32TAmb] -> SM4_Kp/2(sTmSigProces_Te_s32TAmb)
  [rTmComprCtrl_Te_s32TempError] -> SM4_Kp/3(rTmComprCtrl_Te_s32TempError)
  [yTmRefriModeMgr_B_HeatModeInCycle] -> Logical Operator/1
  yTmRefriModeMgr_B_HeatModeInCycle/1 -> [yTmRefriModeMgr_B_HeatModeInCycle]
  [rTmComprCtrl_n_u16DisOverrideValue] -> rSM4_n_u16DisOverrideValue/1
  [rTmComprCtrl_t_u16PIPeriod] -> rSM4_t_u16PIPeriod/1
  [rTmComprCtrl_Te_s32UpErrStop] -> rSM4_Te_s32UpErrStop/1
  [rTmComprCtrl_n_u16ComprRpmFF] -> rSM4_n_u16ComprRpmFF/1
  [rTmComprCtrl_n_u16ComprRpmKp] -> rSM4_n_u16ComprRpmKp/1
  [rTmComprCtrl_Te_s32LowErrStop] -> rSM4_Te_s32LowErrStop/1
  [rTmComprCtrl_n_i16KpUpLimit] -> rSM4_n_i16KpUpLimit/1
  [rTmComprCtrl_n_i16KpLowLimit] -> rSM4_n_i16KpLowLimit/1
  [rTmComprCtrl_n_i16KiUpLimit] -> rSM4_n_i16KiUpLimit/1
  [rTmComprCtrl_n_i16KiLowLimit] -> rSM4_n_i16KiLowLimit/1
  [xTmComprCtrl_B_Enable] -> xSM4_B_Enable/1
  [rTmComprCtrl_n_u16ComprRpmKi] -> rSM4_n_u16ComprRpmKi/1
  [rTmComprCtrl_Te_s32TempError] -> rSM4_Te_s32TempError/1

== system ScriptDemo/Create/createMerge/After/SM5 ==
  note: 20240303
  note: sTmSigProces_Te_s32HvBattCooltTFilter-->sTmSigProces_Te_s32SatLp
  note: sTmIn_Te_s32AmbTEstimd-->sTmSigProces_Te_s32SatLp
  sTmSigProces_Te_s32SatLp : Inport  OutDataTypeStr=single
  sTmSigProces_Te_s32HvBattCooltTFilter : Inport  Port=2  OutDataTypeStr=single
  sTmSigProces_Te_s32HeatrAirTReqRamp : Inport  Port=3  OutDataTypeStr=single
  sTmSigProces_Te_s32HvacHexAirTFilter : Inport  Port=4  OutDataTypeStr=single
  sTmSigProces_Te_s32TempInlet : Inport  Port=5  OutDataTypeStr=single
  sTmSigProces_Te_s32SatHp : Inport  Port=6  OutDataTypeStr=single
  sTmComprCtrl_D_u8HvacFlowLevel : Inport  Port=7  OutDataTypeStr=uint8
  xTmComprCtrl_B_CompOnReqCompOn : Inport  Port=8  OutDataTypeStr=boolean
  yTmHvchCtrl_B_HpcPtcEnad : Inport  Port=9  OutDataTypeStr=boolean
  Action Port : ActionPort
  Constant : Constant  Value=cTmComprCtrl_n_i16SM5CmpHeatKpMax  OutDataTypeStr=int16
  Constant1 : Constant  OutDataTypeStr=boolean
  Constant15 : Constant  Value=cTmComprCtrl_Te_s32ErrCmpPIContinueHeatL  OutDataTypeStr=single
  Constant16 : Constant  Value=cTmComprCtrl_n_i16SM5CmpHeatKiMin  OutDataTypeStr=int16
  Constant17 : Constant  Value=0  OutDataTypeStr=uint16
  Constant6 : Constant  Value=cTmComprCtrl_t_u16SM5CmpHeatPIPeriod  OutDataTypeStr=uint16
  Constant7 : Constant  Value=cTmComprCtrl_n_i16SM5CmpHeatKpMin  OutDataTypeStr=int16
  Constant8 : Constant  Value=cTmComprCtrl_Te_s32ErrCmpPIContinueHeatH  OutDataTypeStr=single
  Constant9 : Constant  Value=cTmComprCtrl_n_i16SM5CmpHeatKiMax  OutDataTypeStr=int16
  ID26291_SM5FF : Subsystem
  ID26293_SM5Error : Subsystem
  SM5FFEnable : Subsystem
  SM5_Ki : Subsystem
  SM5_Kp : Subsystem
  Terminator1 : Terminator
  rSM5_n_u16DisOverrideValue : Outport  OutDataTypeStr=uint16
  rSM5_t_u16PIPeriod : Outport  Port=2  OutDataTypeStr=uint16
  rSM5_Te_s32UpErrStop : Outport  Port=3  OutDataTypeStr=single
  rSM5_n_u16ComprRpmFF : Outport  Port=4  OutDataTypeStr=uint16
  rSM5_n_u16ComprRpmKp : Outport  Port=5  OutDataTypeStr=uint16
  rSM5_Te_s32LowErrStop : Outport  Port=6  OutDataTypeStr=single
  rSM5_n_i16KpUpLimit : Outport  Port=7  OutDataTypeStr=int16
  rSM5_n_i16KpLowLimit : Outport  Port=8  OutDataTypeStr=int16
  rSM5_n_i16KiUpLimit : Outport  Port=9  OutDataTypeStr=int16
  rSM5_n_i16KiLowLimit : Outport  Port=10  OutDataTypeStr=int16
  xSM5_B_Enable : Outport  Port=11  OutDataTypeStr=boolean
  rSM5_n_u16ComprRpmKi : Outport  Port=12  OutDataTypeStr=uint16
  rSM5_Te_s32TempError : Outport  Port=13  OutDataTypeStr=single
  wires:
  ID26293_SM5Error/1(rTmComprCtrl_Te_s32TempError) -> [rTmComprCtrl_Te_s32TempError]
  [sTmSigProces_Te_s32SatHp] -> ID26293_SM5Error/1(sTmSigProces_Te_s32SatHp)
  [yTmHvchCtrl_B_HpcPtcEnad] -> ID26293_SM5Error/2(yTmHvchCtrl_B_HpcPtcEnad)
  [sTmSigProces_Te_s32HeatrAirTReqRamp] -> ID26293_SM5Error/3(sTmSigProces_Te_s32HeatrAirTReqRamp)
  [sTmSigProces_Te_s32HvacHexAirTFilter] -> ID26293_SM5Error/4(sTmSigProces_Te_s32HvacHexAirTFilter)
  sTmSigProces_Te_s32SatLp/1 -> [sTmSigProces_Te_s32SatLp]
  sTmSigProces_Te_s32HvBattCooltTFilter/1 -> Terminator1/1
  sTmSigProces_Te_s32HeatrAirTReqRamp/1 -> [sTmSigProces_Te_s32HeatrAirTReqRamp]
  sTmSigProces_Te_s32HvacHexAirTFilter/1 -> [sTmSigProces_Te_s32HvacHexAirTFilter]
  sTmSigProces_Te_s32TempInlet/1 -> [sTmSigProces_Te_s32TempInlet]
  sTmSigProces_Te_s32SatHp/1 -> [sTmSigProces_Te_s32SatHp]
  sTmComprCtrl_D_u8HvacFlowLevel/1 -> [sTmComprCtrl_D_u8HvacFlowLevel]
  xTmComprCtrl_B_CompOnReqCompOn/1 -> [xTmComprCtrl_B_CompOnReqCompOn]
  yTmHvchCtrl_B_HpcPtcEnad/1 -> [yTmHvchCtrl_B_HpcPtcEnad]
  [xTmComprCtrl_B_CompOnReqCompOn] -> SM5FFEnable/1(xTmComprCtrl_B_CompOnReqCompOn)
  SM5FFEnable/1(SM5FFEnable_B_SM5FFEnable) -> [SM4FFEnable_B_SM4FFEnable]
  [SM4FFEnable_B_SM4FFEnable] -> ID26291_SM5FF/Enable
  ID26291_SM5FF/1(SM5FF) -> [rTmComprCtrl_n_u16ComprRpmFF]
  SM5_Kp/1(SM5Kp) -> [rTmComprCtrl_n_u16ComprRpmKp]
  SM5_Ki/1(SM5Ki) -> [rTmComprCtrl_n_u16ComprRpmKi]
  Constant1/1 -> [xTmComprCtrl_B_Enable]
  Constant16/1 -> [rTmComprCtrl_n_i16KiLowLimit]
  Constant9/1 -> [rTmComprCtrl_n_i16KiUpLimit]
  Constant7/1 -> [rTmComprCtrl_n_i16KpLowLimit]
  Constant8/1 -> [rTmComprCtrl_Te_s32UpErrStop]
  Constant/1 -> [rTmComprCtrl_n_i16KpUpLimit]
  Constant15/1 -> [rTmComprCtrl_Te_s32LowErrStop]
  Constant17/1 -> [rTmComprCtrl_n_u16DisOverrideValue]
  [sTmComprCtrl_D_u8HvacFlowLevel] -> ID26291_SM5FF/1(sTmComprCtrl_D_u8HvacFlowLevel)
  [sTmSigProces_Te_s32TempInlet] -> ID26291_SM5FF/2(sTmSigProces_Te_s32TempInlet)
  [sTmSigProces_Te_s32HeatrAirTReqRamp] -> ID26291_SM5FF/3(sTmSigProces_Te_s32HeatrAirTReqRamp)
  [sTmSigProces_Te_s32SatLp] -> ID26291_SM5FF/4(sTmSigProces_Te_s32SatLp)
  [sTmComprCtrl_D_u8HvacFlowLevel] -> SM5_Ki/1(sTmComprCtrl_D_u8HvacFlowLevel)
  [sTmSigProces_Te_s32SatLp] -> SM5_Ki/2(sTmSigProces_Te_s32SatLp)
  [rTmComprCtrl_Te_s32TempError] -> SM5_Ki/3(rTmComprCtrl_Te_s32TempError)
  [sTmComprCtrl_D_u8HvacFlowLevel] -> SM5_Kp/1(sTmComprCtrl_D_u8HvacFlowLevel)
  [sTmSigProces_Te_s32SatLp] -> SM5_Kp/2(sTmSigProces_Te_s32SatLp)
  [rTmComprCtrl_Te_s32TempError] -> SM5_Kp/3(rTmComprCtrl_Te_s32TempError)
  Constant6/1 -> [rTmComprCtrl_t_u16PIPeriod]
  [rTmComprCtrl_n_u16DisOverrideValue] -> rSM5_n_u16DisOverrideValue/1
  [rTmComprCtrl_t_u16PIPeriod] -> rSM5_t_u16PIPeriod/1
  [rTmComprCtrl_Te_s32UpErrStop] -> rSM5_Te_s32UpErrStop/1
  [rTmComprCtrl_n_u16ComprRpmFF] -> rSM5_n_u16ComprRpmFF/1
  [rTmComprCtrl_n_u16ComprRpmKp] -> rSM5_n_u16ComprRpmKp/1
  [rTmComprCtrl_Te_s32LowErrStop] -> rSM5_Te_s32LowErrStop/1
  [rTmComprCtrl_n_i16KpUpLimit] -> rSM5_n_i16KpUpLimit/1
  [rTmComprCtrl_n_i16KpLowLimit] -> rSM5_n_i16KpLowLimit/1
  [rTmComprCtrl_n_i16KiUpLimit] -> rSM5_n_i16KiUpLimit/1
  [rTmComprCtrl_n_i16KiLowLimit] -> rSM5_n_i16KiLowLimit/1
  [xTmComprCtrl_B_Enable] -> xSM5_B_Enable/1
  [rTmComprCtrl_n_u16ComprRpmKi] -> rSM5_n_u16ComprRpmKi/1
  [rTmComprCtrl_Te_s32TempError] -> rSM5_Te_s32TempError/1

== system ScriptDemo/Create/createMerge/After/SM6 ==
  note: 制热cycle的时候，水回路功能模式为12
  sTmSigProces_Te_s32HeatrAirTReqRamp : Inport  OutDataTypeStr=single
  sTmSigProces_Te_s32HvacHexAirTFilter : Inport  Port=2  OutDataTypeStr=single
  sTmSigProces_Te_s32TempInlet : Inport  Port=3  OutDataTypeStr=single
  sTmSigProces_Te_s32SatHp : Inport  Port=4  OutDataTypeStr=single
  sTmComprCtrl_D_u8HvacFlowLevel : Inport  Port=5  OutDataTypeStr=uint8
  xTmComprCtrl_B_CompOnReqCompOn : Inport  Port=6  OutDataTypeStr=boolean
  yTmHvchCtrl_B_HpcPtcEnad : Inport  Port=7  OutDataTypeStr=boolean
  yTmRefriModeMgr_B_HeatModeInCycle : Inport  Port=8  OutDataTypeStr=boolean
  Action Port : ActionPort
  Constant : Constant  Value=cTmComprCtrl_n_i16SM6CmpHeatKpMax  OutDataTypeStr=int16
  Constant15 : Constant  Value=cTmComprCtrl_Te_s32ErrCmpPIContinueHeatL  OutDataTypeStr=single
  Constant16 : Constant  Value=cTmComprCtrl_n_i16SM6CmpHeatKiMin  OutDataTypeStr=int16
  Constant18 : Constant  Value=cTmComprCtrl_n_i16SM6CmpHeatKiMax  OutDataTypeStr=int16
  Constant2 : Constant  Value=cTmComprCtrl_n_u16CompMinRpm
  Constant7 : Constant  Value=cTmComprCtrl_t_u16SM6CmpHeatPIPeriod  OutDataTypeStr=uint16
  Constant8 : Constant  Value=cTmComprCtrl_n_i16SM6CmpHeatKpMin  OutDataTypeStr=int16
  Constant9 : Constant  Value=cTmComprCtrl_Te_s32ErrCmpPIContinueHeatH  OutDataTypeStr=single
  ID26282_SM6FF : Subsystem
  ID26284_SM6Error : Subsystem
  Logical Operator : Logic  Operator=NOT  AllPortsSameDT=off  OutDataTypeStr=boolean
  SM6FFEnable : Subsystem
  SM6_Ki : Subsystem
  SM6_Kp : Subsystem
  rSM6_n_u16DisOverrideValue : Outport  OutDataTypeStr=uint16
  rSM6_t_u16PIPeriod : Outport  Port=2  OutDataTypeStr=uint16
  rSM6_Te_s32UpErrStop : Outport  Port=3  OutDataTypeStr=single
  rSM6_n_u16ComprRpmFF : Outport  Port=4  OutDataTypeStr=uint16
  rSM6_n_u16ComprRpmKp : Outport  Port=5  OutDataTypeStr=uint16
  rSM6_Te_s32LowErrStop : Outport  Port=6  OutDataTypeStr=single
  rSM6_n_i16KpUpLimit : Outport  Port=7  OutDataTypeStr=int16
  rSM6_n_i16KpLowLimit : Outport  Port=8  OutDataTypeStr=int16
  rSM6_n_i16KiUpLimit : Outport  Port=9  OutDataTypeStr=int16
  rSM6_n_i16KiLowLimit : Outport  Port=10  OutDataTypeStr=int16
  xSM6_B_Enable : Outport  Port=11  OutDataTypeStr=boolean
  rSM6_n_u16ComprRpmKi : Outport  Port=12  OutDataTypeStr=uint16
  rSM6_Te_s32TempError : Outport  Port=13  OutDataTypeStr=single
  wires:
  ID26284_SM6Error/1(rTmComprCtrl_Te_s32TempError) -> [rTmComprCtrl_Te_s32TempError]
  [sTmComprCtrl_D_u8HvacFlowLevel] -> ID26282_SM6FF/1(sTmComprCtrl_D_u8HvacFlowLevel)
  [sTmSigProces_Te_s32TempInlet] -> ID26282_SM6FF/2(sTmSigProces_Te_s32TempInlet)
  [sTmSigProces_Te_s32HeatrAirTReqRamp] -> ID26282_SM6FF/3(sTmSigProces_Te_s32HeatrAirTReqRamp)
  [sTmComprCtrl_D_u8HvacFlowLevel] -> SM6_Ki/1(sTmComprCtrl_D_u8HvacFlowLevel)
  [sTmSigProces_Te_s32TempInlet] -> SM6_Ki/2(sTmSigProces_Te_s32TempInlet)
  [rTmComprCtrl_Te_s32TempError] -> SM6_Ki/3(rTmComprCtrl_Te_s32TempError)
  [sTmComprCtrl_D_u8HvacFlowLevel] -> SM6_Kp/1(sTmComprCtrl_D_u8HvacFlowLevel)
  [sTmSigProces_Te_s32TempInlet] -> SM6_Kp/2(sTmSigProces_Te_s32TempInlet)
  [rTmComprCtrl_Te_s32TempError] -> SM6_Kp/3(rTmComprCtrl_Te_s32TempError)
  [sTmSigProces_Te_s32SatHp] -> ID26284_SM6Error/1(sTmSigProces_Te_s32SatHp)
  [yTmHvchCtrl_B_HpcPtcEnad] -> ID26284_SM6Error/2(yTmHvchCtrl_B_HpcPtcEnad)
  [sTmSigProces_Te_s32HeatrAirTReqRamp] -> ID26284_SM6Error/3(sTmSigProces_Te_s32HeatrAirTReqRamp)
  [sTmSigProces_Te_s32HvacHexAirTFilter] -> ID26284_SM6Error/4(sTmSigProces_Te_s32HvacHexAirTFilter)
  sTmSigProces_Te_s32HeatrAirTReqRamp/1 -> [sTmSigProces_Te_s32HeatrAirTReqRamp]
  sTmSigProces_Te_s32HvacHexAirTFilter/1 -> [sTmSigProces_Te_s32HvacHexAirTFilter]
  sTmSigProces_Te_s32TempInlet/1 -> [sTmSigProces_Te_s32TempInlet]
  sTmSigProces_Te_s32SatHp/1 -> [sTmSigProces_Te_s32SatHp]
  sTmComprCtrl_D_u8HvacFlowLevel/1 -> [sTmComprCtrl_D_u8HvacFlowLevel]
  xTmComprCtrl_B_CompOnReqCompOn/1 -> [xTmComprCtrl_B_CompOnReqCompOn]
  yTmHvchCtrl_B_HpcPtcEnad/1 -> [yTmHvchCtrl_B_HpcPtcEnad]
  ID26282_SM6FF/1(SM6FF) -> [rTmComprCtrl_n_u16ComprRpmFF]
  SM6_Ki/1(SM6Ki) -> [rTmComprCtrl_n_u16ComprRpmKi]
  SM6_Kp/1(SM6Kp) -> [rTmComprCtrl_n_u16ComprRpmKp]
  SM6FFEnable/1(SM6FFEnable_B_SM6FFEnable) -> [SM6FFEnable_B_SM6FFEnable]
  [xTmComprCtrl_B_CompOnReqCompOn] -> SM6FFEnable/1(xTmComprCtrl_B_CompOnReqCompOn)
  [SM6FFEnable_B_SM6FFEnable] -> ID26282_SM6FF/Enable
  Constant/1 -> [rTmComprCtrl_n_i16KpUpLimit]
  Constant2/1 -> [rTmComprCtrl_n_u16DisOverrideValue]
  Constant9/1 -> [rTmComprCtrl_Te_s32UpErrStop]
  Constant8/1 -> [rTmComprCtrl_n_i16KpLowLimit]
  Constant15/1 -> [rTmComprCtrl_Te_s32LowErrStop]
  Constant7/1 -> [rTmComprCtrl_t_u16PIPeriod]
  Constant16/1 -> [rTmComprCtrl_n_i16KiLowLimit]
  Logical Operator/1 -> [xTmComprCtrl_B_Enable]
  Constant18/1 -> [rTmComprCtrl_n_i16KiUpLimit]
  [yTmRefriModeMgr_B_HeatModeInCycle] -> Logical Operator/1
  yTmRefriModeMgr_B_HeatModeInCycle/1 -> [yTmRefriModeMgr_B_HeatModeInCycle]
  [rTmComprCtrl_n_u16DisOverrideValue] -> rSM6_n_u16DisOverrideValue/1
  [rTmComprCtrl_t_u16PIPeriod] -> rSM6_t_u16PIPeriod/1
  [rTmComprCtrl_Te_s32UpErrStop] -> rSM6_Te_s32UpErrStop/1
  [rTmComprCtrl_n_u16ComprRpmFF] -> rSM6_n_u16ComprRpmFF/1
  [rTmComprCtrl_n_u16ComprRpmKp] -> rSM6_n_u16ComprRpmKp/1
  [rTmComprCtrl_Te_s32LowErrStop] -> rSM6_Te_s32LowErrStop/1
  [rTmComprCtrl_n_i16KpUpLimit] -> rSM6_n_i16KpUpLimit/1
  [rTmComprCtrl_n_i16KpLowLimit] -> rSM6_n_i16KpLowLimit/1
  [rTmComprCtrl_n_i16KiUpLimit] -> rSM6_n_i16KiUpLimit/1
  [rTmComprCtrl_n_i16KiLowLimit] -> rSM6_n_i16KiLowLimit/1
  [xTmComprCtrl_B_Enable] -> xSM6_B_Enable/1
  [rTmComprCtrl_n_u16ComprRpmKi] -> rSM6_n_u16ComprRpmKi/1
  [rTmComprCtrl_Te_s32TempError] -> rSM6_Te_s32TempError/1

== system ScriptDemo/Create/createMerge/After/SM7 ==
  sTmSigProces_Te_s32TAmb : Inport  OutDataTypeStr=single
  sTmSigProces_Te_s32HvBattCooltTOutFilter : Inport  Port=2  OutDataTypeStr=single
  Action Port : ActionPort
  2-D Lookup Table11 : Lookup_n-D  LookupTableObject=mTmComprCtrl_n_u16FFCmpSpdChillDeice  BreakpointsForDimension1=mTmComprCtrl_n_u16FFCmpSpdChillDeice_Y  BreakpointsForDimension2=mTmComprCtrl_n_u16FFCmpSpdChillDeice_X  BreakpointsForDimension1DataTypeStr=Inherit: Inherit from 'Breakpoint data'  BreakpointsForDimension2DataTypeStr=Inherit: Inherit from 'Breakpoint data'  Table=mTmComprCtrl_n_u16FFCmpSpdChillDeice  TableDataTypeStr=Inherit: Inherit from 'Table data'  ExtrapMethod=Clip  InternalRulePriority=Speed  OutDataTypeStr=Inherit: Inherit via back propagation  RndMeth=Simplest  InputSameDT=off
      settings: InputPortMap=u0,u1
  Constant : Constant  Value=0  OutDataTypeStr=uint16
  Constant1 : Constant  Value=0  OutDataTypeStr=uint16
  Constant11 : Constant  Value=5  OutDataTypeStr=uint16
  Constant12 : Constant  Value=0  OutDataTypeStr=boolean
  Constant2 : Constant  Value=0  OutDataTypeStr=uint16
  Constant3 : Constant  Value=0  OutDataTypeStr=single
  Constant4 : Constant  Value=0  OutDataTypeStr=single
  Constant5 : Constant  Value=0  OutDataTypeStr=single
  Constant{6..9} (4 alike) : Constant  Value=0  OutDataTypeStr=int16
  rSM7_n_u16DisOverrideValue : Outport  OutDataTypeStr=uint16
  rSM7_t_u16PIPeriod : Outport  Port=2  OutDataTypeStr=uint16
  xSM7_B_Enable : Outport  Port=3  OutDataTypeStr=boolean
  rSM7_n_i16KiUpLimit : Outport  Port=4  OutDataTypeStr=int16
  rSM7_n_i16KiLowLimit : Outport  Port=5  OutDataTypeStr=int16
  rSM7_Te_s32TempError : Outport  Port=6  OutDataTypeStr=single
  rSM7_n_u16ComprRpmFF : Outport  Port=7  OutDataTypeStr=uint16
  rSM7_n_u16ComprRpmKp : Outport  Port=8  OutDataTypeStr=uint16
  rSM7_n_u16ComprRpmKi : Outport  Port=9  OutDataTypeStr=uint16
  rSM7_Te_s32UpErrStop : Outport  Port=10  OutDataTypeStr=single
  rSM7_Te_s32LowErrStop : Outport  Port=11  OutDataTypeStr=single
  rSM7_n_i16KpUpLimit : Outport  Port=12  OutDataTypeStr=int16
  rSM7_n_i16KpLowLimit : Outport  Port=13  OutDataTypeStr=int16
  wires:
  [sTmSigProces_Te_s32TAmb] -> 2-D Lookup Table11/2
  [sTmSigProces_Te_s32HvBattCooltTOutFilter] -> 2-D Lookup Table11/1
  sTmSigProces_Te_s32TAmb/1 -> [sTmSigProces_Te_s32TAmb]
  sTmSigProces_Te_s32HvBattCooltTOutFilter/1 -> [sTmSigProces_Te_s32HvBattCooltTOutFilter]
  2-D Lookup Table11/1 -> [rTmComprCtrl_n_u16DisOverrideValue]
  Constant12/1 -> [xTmComprCtrl_B_Enable]
  Constant7/1 -> [rTmComprCtrl_n_i16KiUpLimit]
  Constant8/1 -> [rTmComprCtrl_n_i16KiLowLimit]
  Constant11/1 -> [rTmComprCtrl_t_u16PIPeriod]
  Constant5/1 -> [rTmComprCtrl_Te_s32LowErrStop]
  Constant/1 -> [rTmComprCtrl_n_u16ComprRpmFF]
  Constant6/1 -> [rTmComprCtrl_n_i16KpLowLimit]
  Constant1/1 -> [rTmComprCtrl_n_u16ComprRpmKp]
  Constant9/1 -> [rTmComprCtrl_n_i16KpUpLimit]
  Constant2/1 -> [rTmComprCtrl_n_u16ComprRpmKi]
  Constant4/1 -> [rTmComprCtrl_Te_s32TempError]
  Constant3/1 -> [rTmComprCtrl_Te_s32UpErrStop]
  [rTmComprCtrl_n_u16DisOverrideValue] -> rSM7_n_u16DisOverrideValue/1
  [rTmComprCtrl_t_u16PIPeriod] -> rSM7_t_u16PIPeriod/1
  [xTmComprCtrl_B_Enable] -> xSM7_B_Enable/1
  [rTmComprCtrl_n_i16KiUpLimit] -> rSM7_n_i16KiUpLimit/1
  [rTmComprCtrl_n_i16KiLowLimit] -> rSM7_n_i16KiLowLimit/1
  [rTmComprCtrl_Te_s32TempError] -> rSM7_Te_s32TempError/1
  [rTmComprCtrl_n_u16ComprRpmFF] -> rSM7_n_u16ComprRpmFF/1
  [rTmComprCtrl_n_u16ComprRpmKp] -> rSM7_n_u16ComprRpmKp/1
  [rTmComprCtrl_n_u16ComprRpmKi] -> rSM7_n_u16ComprRpmKi/1
  [rTmComprCtrl_Te_s32UpErrStop] -> rSM7_Te_s32UpErrStop/1
  [rTmComprCtrl_Te_s32LowErrStop] -> rSM7_Te_s32LowErrStop/1
  [rTmComprCtrl_n_i16KpUpLimit] -> rSM7_n_i16KpUpLimit/1
  [rTmComprCtrl_n_i16KpLowLimit] -> rSM7_n_i16KpLowLimit/1
